simulink model "NMC_Cell_model"  (R2022a)
settings: Solver=VariableStepAuto  StartTime=0.0  StopTime=60  MaxStep=0.01  RelTol=1e-3
settings Model: Creator=matm  LastModifiedBy=nikos
settings SolverCC: ShapePreserveControl=EnableAll  AlgebraicLoopSolver=TrustRegion  SolverResetMethod=Robust
settings DataIOCC: ReturnWorkspaceOutputs=off
settings DebuggingCC: UnconnectedInputMsg=warning  UnconnectedOutputMsg=warning  UnconnectedLineMsg=warning  SFMachineParentedDataDiag=warning  ArithmeticOperatorsInVariantConditions=warning
settings SFSimCC: SimUseLocalCustomCode=off  CustomCodeUndefinedFunction=UseInterfaceOnly
settings RTWCC: RTWUseLocalCustomCode=off  DLArmComputeVersion=19.05
settings CodeAppCC: StateflowObjectComments=on

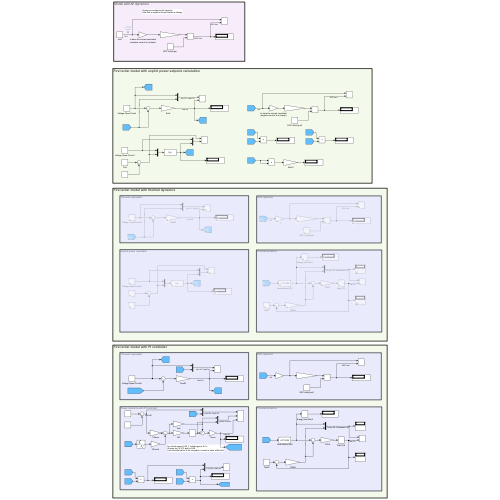
[thumbnail: Simulink's stored preview of the top-level diagram]
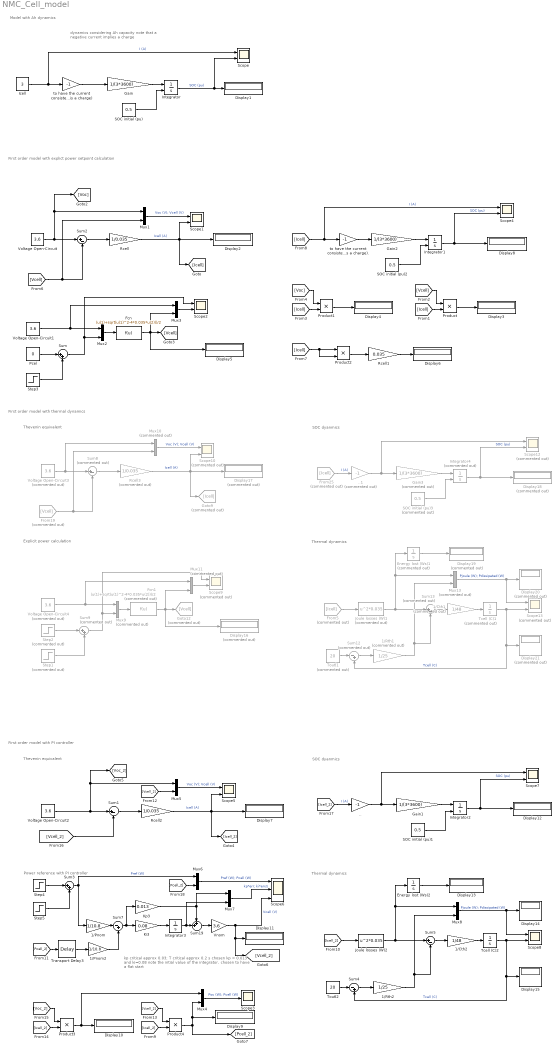
== system NMC_Cell_model ==
  note: Explicit power calculation
  note: First order model with explict power setpoint calculation
  note: Model with Ah dynamics
  note: dynamics considering Ah capacity
      | note that a negative current implies a charge
  note: Thermal dynamics
  note: Power reference with PI controller
  note: Thevenin equivalent
  note: SOC dyanmics
  note: First order model with PI controller
  note: kp critical approx 0.03; T critical approx 0.2 s
      | chosen kp = 0.013 and ki=0.08
      | note the intial value of the integrator, chosen to have a flat start
  note: Thevenin equivalent
  note: Thermal dynamics
  note: SOC dyanmics
  note: First order model with thermal dynamics
  .. : Gain  Gain=-1
  ..1 : Gain  Commented=on  Gain=-1
  1/Cth1 : Gain  Commented=on  Gain=1/48
  1/Cth2 : Gain  Gain=1/48
  1/Pnom : Gain  Gain=1/10.8
  1/Pnom2 : Gain  Gain=1/10.8
  1/Rth1 : Gain  Commented=on  Gain=1/25
  1/Rth2 : Gain  Gain=1/25
  Display{1..15} (15 alike) : Display
  Display{16..21} (6 alike) : Display  Commented=on
  Energy lost (Ws)1 : Integrator  Commented=on  ZeroCross=off
  Energy lost (Ws)2 : Integrator  ZeroCross=off
  Fcn : Fcn  Expr=(u(1)+sqrt(u(1)^2-4*0.035*u(2)))/2
  Fcn1 : Fcn  Commented=on  Expr=(u(1)+sqrt(u(1)^2-4*0.035*u(2)))/2
  From19 : From  Commented=on  GotoTag=Vcell
  From25 : From  Commented=on  GotoTag=Icell
  From5 : From  Commented=on  GotoTag=Icell
  Gain : Gain  Gain=1/(3*3600)
  Gain1 : Gain  Gain=1/(3*3600)
  Gain2 : Gain  Gain=1/(3*3600)
  Gain3 : Gain  Commented=on  Gain=1/(3*3600)
  Goto12 : Goto  Commented=on  GotoTag=Vcell
  Goto9 : Goto  Commented=on  GotoTag=Icell
  Icell : Constant  Value=3
  Integrator : Integrator  InitialConditionSource=external  InitialCondition=0.5  UpperSaturationLimit=1  ZeroCross=off
  Integrator1 : Integrator  InitialConditionSource=external  InitialCondition=0.5  ZeroCross=off
  Integrator2 : Integrator  InitialConditionSource=external  InitialCondition=0.5  ZeroCross=off
  Integrator3 : Integrator  InitialCondition=1  ZeroCross=off
  Integrator4 : Integrator  Commented=on  InitialConditionSource=external  InitialCondition=0.5  ZeroCross=off
  Joule losses (W)1 : Fcn  Commented=on  Expr=u^2*0.035
  Joule losses (W)2 : Fcn  Expr=u^2*0.035
  Ki3 : Gain  Gain=0.08
  Kp3 : Gain  Gain=0.013
  Mux{1..8} (8 alike) : Mux  Inputs=2
  Mux{9..11,13} (4 alike) : Mux  Commented=on  Inputs=2
  Pcel : Constant  Value=0
  Product{,1..4} (5 alike) : Product
  Rcell : Gain  Gain=1/0.035
  Rcell1 : Gain  Gain=0.035
  Rcell2 : Gain  Gain=1/0.035
  Rcell3 : Gain  Commented=on  Gain=1/0.035
  SOC initial (pu) : Constant  Value=0.5
  SOC initial (pu)1 : Constant  Value=0.5
  SOC initial (pu)2 : Constant  Value=0.5
  SOC initial (pu)3 : Constant  Commented=on  Value=0.5
  Scope{,1..2,4..5,7..8} (7 alike) : Scope  NumInputPorts=2
  Scope{9..10,12..13} (4 alike) : Scope  Commented=on  NumInputPorts=2
  Scope3 : Scope
  Scope6 : Scope  NumInputPorts=3
  Step1 : Step  Commented=on  Time=1210  After=-10.8  SampleTime=0
  Step2 : Step  Commented=on  Time=10  After=10.8  SampleTime=0
  Step3 : Step  After=10.8  SampleTime=0
  Step4 : Step  Time=10  After=10.8  SampleTime=0
  Step5 : Step  Time=610  After=-10.8  SampleTime=0
  Sum : Sum  Inputs=|++
  Sum1 : Sum  Inputs=|+-
  Sum12 : Sum  Commented=on  Inputs=|-+
  Sum13 : Sum  Commented=on  Inputs=|+-
  Sum19 : Sum  Inputs=++|
  Sum2 : Sum  Inputs=|+-
  Sum3 : Sum  Inputs=|++
  Sum4 : Sum  Inputs=|-+
  Sum5 : Sum  Inputs=|+-
  Sum7 : Sum  Inputs=|-+
  Sum8 : Sum  Commented=on  Inputs=|+-
  Sum9 : Sum  Commented=on  Inputs=|++
  Tcell (C)1 : Integrator  Commented=on  InitialCondition=20  ZeroCross=off
  Tcell (C)2 : Integrator  InitialCondition=20  ZeroCross=off
  Toutl1 : Constant  Commented=on  Value=20
  Toutl2 : Constant  Value=20
  Transport Delay3 : TransportDelay  DelayTime=0.1
  Vnom : Gain  Gain=3.6
  Voltage Open-Circuit : Constant  Value=3.6
  Voltage Open-Circuit1 : Constant  Value=3.6
  Voltage Open-Circuit2 : Constant  Value=3.6
  Voltage Open-Circuit3 : Constant  Commented=on  Value=3.6
  Voltage Open-Circuit4 : Constant  Commented=on  Value=3.6
  to have the current consistent (negative current is a charge) : Gain  Gain=-1
  to have the current consistent (negative current is a charge). : Gain  Gain=-1
  wires:
  Integrator/1 -> Display1/1, Scope/2  "SOC (pu)"
  Gain/1 -> Integrator/1
  Icell/1 -> Scope/1, to have the current consistent (negative current is a charge)/1  "I (A)"
  Voltage Open-Circuit/1 -> [Voc], Mux1/1, Sum2/1
  [Vcell] -> Mux1/2, Sum2/2
  Sum2/1 -> Rcell/1
  Mux1/1 -> Scope1/1  "Voc (V); Vcell (V)"
  Rcell/1 -> [Icell], Scope1/2, Display2/1  "Icell (A)"
  SOC initial (pu)/1 -> Integrator/2
  [Icell] -> Product/2
  Product/1 -> Display3/1
  [Vcell] -> Product/1
  [Icell] -> Product1/2
  Product1/1 -> Display4/1
  [Voc] -> Product1/1
  Mux2/1 -> Fcn/1
  Voltage Open-Circuit1/1 -> Mux2/1, Mux3/1
  Fcn/1 -> Display5/1, Mux3/2, [Vcell]
  Mux3/1 -> Scope2/2
  [Icell] -> Product2/2, Product2/1
  Product2/1 -> Rcell1/1
  Rcell1/1 -> Display6/1
  to have the current consistent (negative current is a charge)/1 -> Gain/1
  Gain2/1 -> Integrator1/1
  to have the current consistent (negative current is a charge)./1 -> Gain2/1
  [Icell] -> Scope4/1, to have the current consistent (negative current is a charge)./1  "I (A)"
  SOC initial (pu)2/1 -> Integrator1/2
  Integrator1/1 -> Scope4/2, Display8/1  "SOC (pu)"
  [Icell_2] -> ../1  "I (A)"
  SOC initial (pu)1/1 -> Integrator2/2
  Energy lost (Ws)2/1 -> Display13/1
  Rcell2/1 -> [Icell_2], Scope5/2, Display7/1  "Icell (A)"
  [Voc_2] -> Product3/1
  Step4/1 -> Sum3/1
  [Vcell_2] -> Product4/1
  Sum4/1 -> 1/Rth2/1
  [Icell_2] -> Product4/2
  Product3/1 -> Mux4/1, Display10/1
  [Icell_2] -> Joule losses (W)2/1
  Sum5/1 -> 1/Cth2/1
  1/Rth2/1 -> Sum5/2, Mux8/2
  Integrator2/1 -> Scope7/2, Display12/1  "SOC (pu)"
  Joule losses (W)2/1 -> Sum5/1, Energy lost (Ws)2/1, Mux8/1
  Sum3/1 -> Mux6/1, 1/Pnom/1  "Pref (W)"
  Mux5/1 -> Scope5/1  "Voc (V); Vcell (V)"
  Voltage Open-Circuit2/1 -> [Voc_2], Mux5/1, Sum1/1
  Mux6/1 -> Scope6/1  "Pref (W); Pcell (W)"
  [Vcell_2] -> Mux5/2
  Toutl2/1 -> Sum4/1
  Mux8/1 -> Display14/1, Scope8/1  "Pjoule (W); Pdissipated (W)"
  Vnom/1 -> Scope6/3, [Vcell_2], Display11/1  "Vcell (V)"
  Ki3/1 -> Integrator3/1
  Integrator3/1 -> Mux7/2, Sum19/2
  1/Cth2/1 -> Tcell (C)2/1
  Sum1/1 -> Rcell2/1
  Mux7/1 -> Scope6/2  "kp*err; ki*err/s"
  Gain1/1 -> Integrator2/1
  1/Pnom/1 -> Sum7/1
  Mux4/1 -> Scope3/1  "Poc (W); Pcell (W)"
  Kp3/1 -> Mux7/1, Sum19/1
  Sum7/1 -> Kp3/1, Ki3/1
  ../1 -> Scope7/1, Gain1/1
  [Pcell_2] -> Mux6/2
  Product4/1 -> Mux4/2, Display9/1, [Pcell_2]
  1/Pnom2/1 -> Sum7/2
  [Pcell_2] -> Transport Delay3/1
  Tcell (C)2/1 -> Scope8/2, Display15/1, Sum4/2  "Tcell (C)"
  [Icell_2] -> Product3/2
  Step5/1 -> Sum3/2
  Sum19/1 -> Vnom/1
  Transport Delay3/1 -> 1/Pnom2/1
  Integrator4/1 -> Scope12/2, Display18/1  "SOC (pu)"
  Joule losses (W)1/1 -> Sum13/1, Energy lost (Ws)1/1, Mux13/1
  1/Rth1/1 -> Sum13/2, Mux13/2
  From5/1 -> Joule losses (W)1/1
  Sum13/1 -> 1/Cth1/1
  Energy lost (Ws)1/1 -> Display19/1
  From25/1 -> ..1/1  "I (A)"
  ..1/1 -> Scope12/1, Gain3/1
  SOC initial (pu)3/1 -> Integrator4/2
  Gain3/1 -> Integrator4/1
  1/Cth1/1 -> Tcell (C)1/1
  Mux13/1 -> Display20/1, Scope13/1  "Pjoule (W); Pdissipated (W)"
  Tcell (C)1/1 -> Scope13/2, Display21/1, Sum12/2  "Tcell (C)"
  Toutl1/1 -> Sum12/1
  Sum12/1 -> 1/Rth1/1
  Mux9/1 -> Fcn1/1
  Step2/1 -> Sum9/1
  Mux11/1 -> Scope9/2
  Step1/1 -> Sum9/2
  Voltage Open-Circuit4/1 -> Mux9/1, Mux11/1
  Sum9/1 -> Mux9/2, Scope9/1
  Fcn1/1 -> Display16/1, Mux11/2, Goto12/1
  From19/1 -> Mux10/2, Sum8/2
  Rcell3/1 -> Goto9/1, Scope10/2, Display17/1  "Icell (A)"
  Sum8/1 -> Rcell3/1
  Mux10/1 -> Scope10/1  "Voc (V); Vcell (V)"
  Voltage Open-Circuit3/1 -> Mux10/1, Sum8/1
  Pcel/1 -> Sum/1
  Sum/1 -> Scope2/1, Mux2/2
  Step3/1 -> Sum/2
  [Vcell_2] -> Sum1/2
